simulink model "Non-coherent demodulator"  (R2022a)
settings: Solver=FixedStepAuto  StartTime=0.0  StopTime=50e-3  FixedStep=1e-6  RelTol=1e-3
libraries: dspsrcs4 x4, dsparch4 x1
settings Model: Creator=Camille  LastModifiedBy=Camille

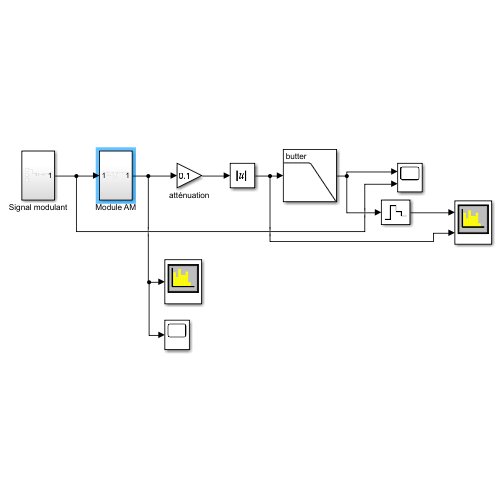
[thumbnail: Simulink's stored preview of the top-level diagram]
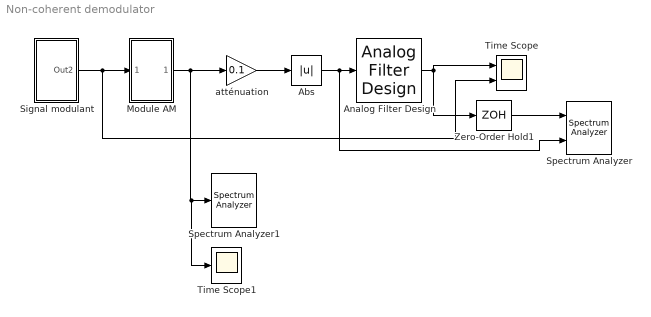
== system Non-coherent demodulator ==
  Abs : Abs  SaturateOnIntegerOverflow=off
  Analog Filter Design : dsparch4/Analog Filter Design  method=Butterworth  filttype=Lowpass  N=8  Wlo=70000  Whi=80  Rp=2  Rs=40
  Module AM : Subsystem
  Signal modulant : Subsystem
  Spectrum Analyzer : SpectrumAnalyzer  NumInputPorts=2
  Spectrum Analyzer1 : SpectrumAnalyzer
  Time Scope : Scope  NumInputPorts=2
  Time Scope1 : Scope
  Zero-Order Hold1 : ZeroOrderHold  SampleTime=1e-6
  atténuation : Gain  Gain=0.1
  wires:
  Signal modulant/1(Out2) -> Time Scope/2, Module AM/1(In1)
  Abs/1 -> Analog Filter Design/1, Spectrum Analyzer/2
  Analog Filter Design/1 -> Time Scope/1, Zero-Order Hold1/1
  Zero-Order Hold1/1 -> Spectrum Analyzer/1
  Module AM/1(Out1) -> Time Scope1/1, Spectrum Analyzer1/1, atténuation/1
  atténuation/1 -> Abs/1

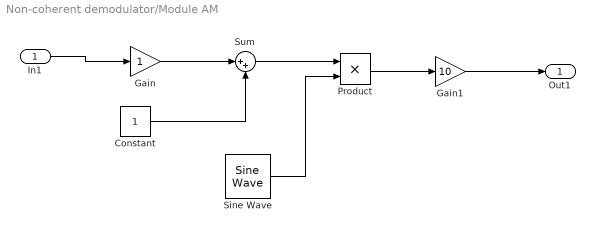
== system Non-coherent demodulator/Module AM ==
  In1 : Inport
  Constant : Constant
  Gain : Gain
  Gain1 : Gain  Gain=10
  Product : Product
  Sine Wave : dspsrcs4/Sine Wave  Amplitude=1  Frequency=20e3  Phase=pi/2  SampleMode=Discrete  OutComplex=Real  CompMethod=Trigonometric fcn  TableSize=Speed  SampleTime=0.1e-5  SamplesPerFrame=1  ResetState=Restart at time zero  OutputFrames=off  dataType=double  wordLen=16  udDataType=sfix(16)  fracBitsMode=Best precision  numFracBits=15  OutDataTypeStr=double  LastOutDataTypeStr=double
  Sum : Sum  Inputs=|++
  Out1 : Outport
  wires:
  Gain/1 -> Sum/1
  Gain1/1 -> Out1/1
  Constant/1 -> Sum/2
  Sine Wave/1 -> Product/2
  Sum/1 -> Product/1
  In1/1 -> Gain/1
  Product/1 -> Gain1/1

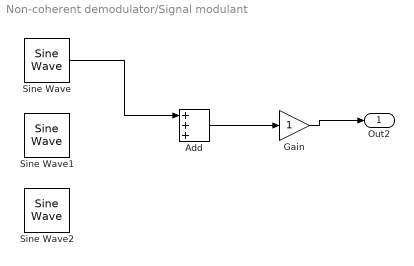
== system Non-coherent demodulator/Signal modulant ==
  Add : Sum  Inputs=+++
  Gain : Gain
  Sine Wave : dspsrcs4/Sine Wave  Amplitude=1  Frequency=0.5e3  Phase=0  SampleMode=Discrete  OutComplex=Real  CompMethod=Trigonometric fcn  TableSize=Speed  SampleTime=1e-6  SamplesPerFrame=1  ResetState=Restart at time zero  OutputFrames=off  dataType=double  wordLen=16  udDataType=sfix(16)  fracBitsMode=Best precision  numFracBits=15  OutDataTypeStr=double  LastOutDataTypeStr=double
  Sine Wave1 : dspsrcs4/Sine Wave  Amplitude=0.5  Frequency=1.5e3  Phase=0  SampleMode=Discrete  OutComplex=Real  CompMethod=Trigonometric fcn  TableSize=Speed  SampleTime=1e-6  SamplesPerFrame=1  ResetState=Restart at time zero  OutputFrames=off  dataType=double  wordLen=16  udDataType=sfix(16)  fracBitsMode=Best precision  numFracBits=15  OutDataTypeStr=double  LastOutDataTypeStr=double
  Sine Wave2 : dspsrcs4/Sine Wave  Amplitude=0.2  Frequency=2.5e3  Phase=0  SampleMode=Discrete  OutComplex=Real  CompMethod=Trigonometric fcn  TableSize=Speed  SampleTime=1e-6  SamplesPerFrame=1  ResetState=Restart at time zero  OutputFrames=off  dataType=double  wordLen=16  udDataType=sfix(16)  fracBitsMode=Best precision  numFracBits=15  OutDataTypeStr=double  LastOutDataTypeStr=double
  Out2 : Outport
  wires:
  Add/1 -> Gain/1
  Gain/1 -> Out2/1
  Sine Wave/1 -> Add/1
